simulink model "newmodel"  (R2023a)
settings: Solver=VariableStepAuto  StartTime=0.0  StopTime=10.0  RelTol=1e-3
values from neighbouring files (symbols this model uses):
  C_M = 1.3    [newconst.m]
  C_W = 3.15    [newconst.m]
  J_mot = 7*10^-6    (= 7e-06)    [newconst.m]
  L_a = 0.0015    [newconst.m]
  L_fw = 0.013    [newconst.m]
  R_a = 8    [newconst.m]
settings Model: Creator=79056  LastModifiedBy=79056

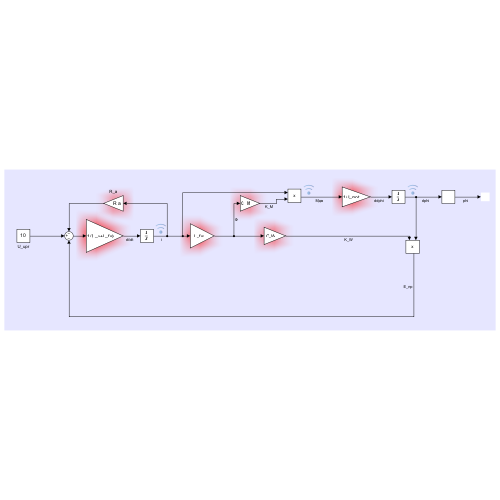
[thumbnail: Simulink's stored preview of the top-level diagram]
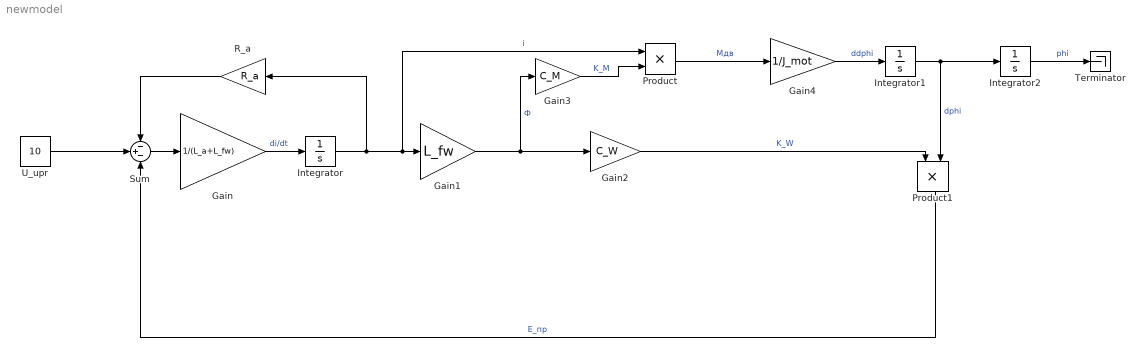
== system newmodel ==
  Gain : Gain  Gain=1/(L_a+L_fw)
  Gain1 : Gain  Gain=L_fw
  Gain2 : Gain  Gain=C_W
  Gain3 : Gain  Gain=C_M
  Gain4 : Gain  Gain=1/J_mot
  Integrator : Integrator
  Integrator1 : Integrator
  Integrator2 : Integrator
  Product : Product
  Product1 : Product
  R_a : Gain  Gain=R_a
  Sum : Sum  Inputs=-+-
  Terminator : Terminator
  U_upr : Constant  Value=10
  wires:
  Gain3/1 -> Product/2  "K_M"
  Integrator1/1 -> Product1/2, Integrator2/1  "dphi"
  Integrator2/1 -> Terminator/1  "phi"
  U_upr/1 -> Sum/2
  Gain4/1 -> Integrator1/1  "ddphi"
  R_a/1 -> Sum/1
  Integrator/1 -> Product/1, Gain1/1, R_a/1  "i"
  Product/1 -> Gain4/1  "Mдв"
  Gain1/1 -> Gain3/1, Gain2/1  "Ф"
  Gain2/1 -> Product1/1  "K_W"
  Gain/1 -> Integrator/1  "di/dt"
  Product1/1 -> Sum/3  "E_пр"
  Sum/1 -> Gain/1
